simulink model "sim_cont_est_2022b"  (R2022b)
settings: Solver=FixedStepAuto  StartTime=0.0  StopTime=10.0  FixedStep=0.05  RelTol=1e-3
values from neighbouring files (symbols this model uses):
  A = 208.220778648    [estimated_AB.mat]
  B = 20.4160211826    [estimated_AB.mat]
libraries: mpclib x1
settings Model: Creator=RAOUF  LastModifiedBy=Claudia Yasar
settings DataIOCC: ReturnWorkspaceOutputs=off
settings OptimizationCC: ReuseModelBlockBuffer=on

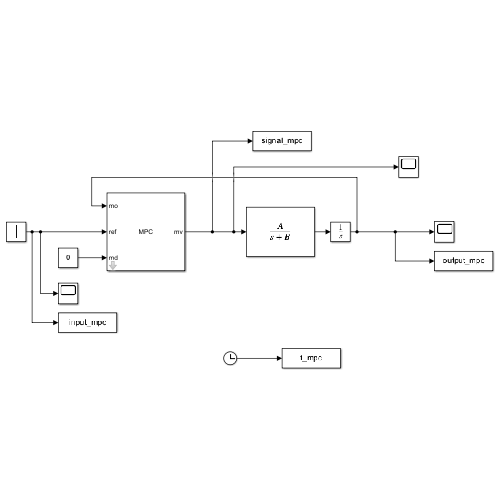
[thumbnail: Simulink's stored preview of the top-level diagram]
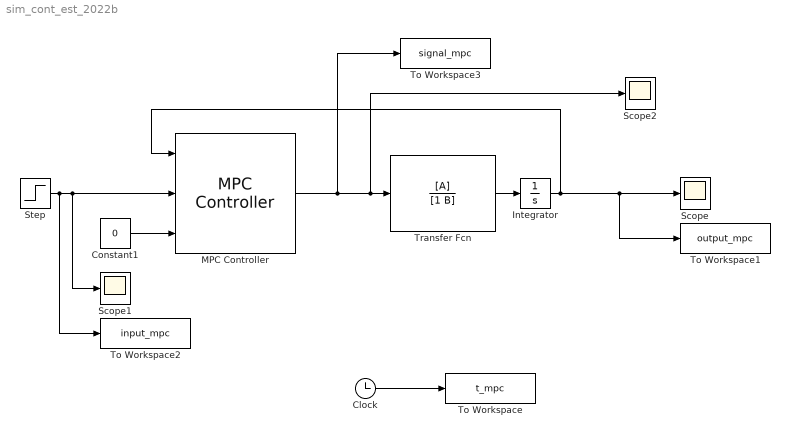
== system sim_cont_est_2022b ==
  Clock : Clock
  Constant1 : Constant  Value=0
  Integrator : Integrator
  MPC Controller : mpclib/MPC Controller  SCDEnableBlockLinearizationSpecification=on  mpcobj=mpc1  is_multiple=0  enable_value=0  return_u0=off  updateMPCinCallerWorkspace=on  md_inport=on  mv_inport=off  uref_inport=off  return_cost=off  return_mvseq=off  return_qpstatus=off  return_xseq=off  return_state=off  return_ovseq=off  state_inport=off  umin_inport=off  umax_inport=off  ymin_inport=off  ymax_inport=off  cc_inport=off  ywt_inport=off  uwt_inport=off  duwt_inport=off  rhoeps_inport=off  pm_inport=off  MaximumP=10  HorizonChoice=FixedHorizon  n_ts=0.05  n_p=10  n_mv=1  n_md=1  n_ud=0  n_mo=1  n_uo=0  BlockDataType=double  SampleTimeInherited=off  switch_inport=off
  Scope : Scope
  Scope1 : Scope
  Scope2 : Scope
  Step : Step  After=pi/2  SampleTime=0
  To Workspace : ToWorkspace  VariableName=t_mpc  SampleTime=-1
      settings: Save2DSignal=2-D array (concatenate along first dimension)
  To Workspace1 : ToWorkspace  VariableName=output_mpc  SampleTime=-1
      settings: Save2DSignal=2-D array (concatenate along first dimension)
  To Workspace2 : ToWorkspace  VariableName=input_mpc  SampleTime=-1
      settings: Save2DSignal=2-D array (concatenate along first dimension)
  To Workspace3 : ToWorkspace  VariableName=signal_mpc  SampleTime=-1
      settings: Save2DSignal=2-D array (concatenate along first dimension)
  Transfer Fcn : TransferFcn  Numerator=[A]  Denominator=[1 B]
  wires:
  Constant1/1 -> MPC Controller/3
  Transfer Fcn/1 -> Integrator/1
  Integrator/1 -> To Workspace1/1, Scope/1, MPC Controller/1
  Clock/1 -> To Workspace/1
  Step/1 -> MPC Controller/2, Scope1/1, To Workspace2/1
  MPC Controller/1 -> To Workspace3/1, Scope2/1, Transfer Fcn/1
